simulink model "P_model"  (R2018b)
settings: Solver=VariableStepAuto  StartTime=0.0  StopTime=10.0  RelTol=1e-3
undefined symbols (not defined in the file or in its folder): alpha
settings Model: Creator=rache  LastModifiedBy=rache

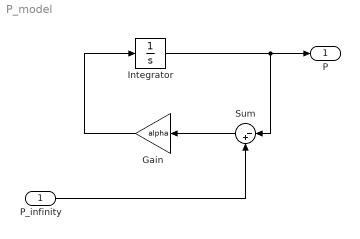
== system P_model ==
  P_infinity : Inport
  Gain : Gain  Gain=alpha
  Integrator : Integrator
  Sum : Sum  Inputs=|-+
  P : Outport
  wires:
  Sum/1 -> Gain/1
  P_infinity/1 -> Sum/2
  Integrator/1 -> P/1, Sum/1
  Gain/1 -> Integrator/1
